simulink model "CH22_3A"  (Simulink 7.5)
settings: Solver=ode45  StartTime=0.0  StopTime=20  RelTol=1e-3
libraries: commrandsrc2 x2, commutil2 x2, commfilt2 x1
settings Model: Creator=my2  LastModifiedBy=xnote
settings OptimizationCC: ExpressionDepthLimit=128
settings DebuggingCC: MultiTaskDSMMsg=warning  MultiTaskCondExecSysMsg=none  StateNameClashWarn=none  StrictBusMsg=None
settings RTWCC: IncludeERTFirstTime=on
settings CodeAppCC: CustomSymbolStrType=$N$R$M_T
settings GRTTargetCC: CombineOutputUpdateFcns=on  CPPClassGenCompliant=on

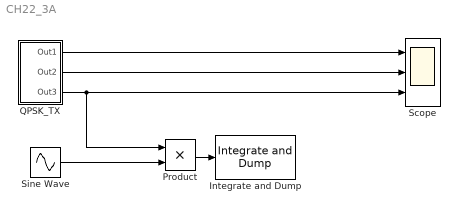
== system CH22_3A ==
  Integrate and Dump : commfilt2/Integrate and Dump  DialogController=commDDGCreate  DialogControllerArgs=DataTag0  obssamples=8  offsetsamples=0  nodump=off  roundingMode=Floor  overflowMode=off
  Product : Product
  QPSK_TX : Subsystem
  Scope : Scope  NumInputPorts=3
      settings: YMin=-5~-5~-5  YMax=5~5~5
  Sine Wave : Sin  Amplitude=1  Bias=0  Frequency=1  Phase=0  Samples=10  SampleTime=1/256  Offset=0
  wires:
  QPSK_TX/1(Out1) -> Scope/1
  QPSK_TX/2(Out2) -> Scope/2
  QPSK_TX/3(Out3) -> Product/1, Scope/3
  Sine Wave/1 -> Product/2
  Product/1 -> Integrate and Dump/1

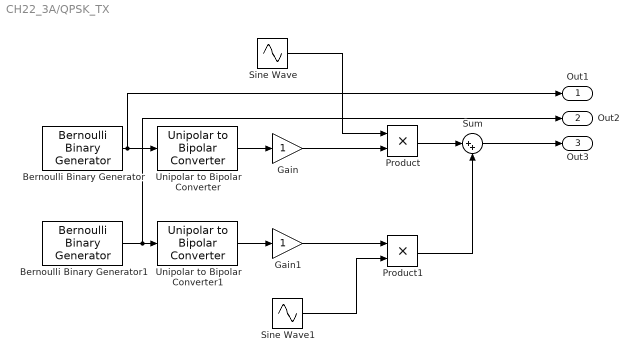
== system CH22_3A/QPSK_TX ==
  Bernoulli Binary Generator : commrandsrc2/Bernoulli Binary Generator  DialogController=commDDGCreate  DialogControllerArgs=DataTag1  SystemSampleTime=-1  P=0.5  seed=71  Ts=1  frameBased=off  sampPerFrame=1  orient=off  outDataType=boolean
  Bernoulli Binary Generator1 : commrandsrc2/Bernoulli Binary Generator  DialogController=commDDGCreate  DialogControllerArgs=DataTag2  SystemSampleTime=-1  P=0.5  seed=61  Ts=1  frameBased=off  sampPerFrame=1  orient=off  outDataType=boolean
  Gain : Gain
  Gain1 : Gain
  Product : Product
  Product1 : Product
  Sine Wave : Sin  Amplitude=1  Bias=0  Frequency=1  Phase=0  Samples=10  SampleTime=1/256  Offset=0
  Sine Wave1 : Sin  Amplitude=1  Bias=0  Frequency=1  Phase=0  Samples=10  SampleTime=1/256  Offset=0
  Sum : Sum  Inputs=|++
  Unipolar to Bipolar Converter : commutil2/Unipolar to Bipolar Converter  SystemSampleTime=-1  M=2  polarity=Positive  dataType=Inherit via internal rule
  Unipolar to Bipolar Converter1 : commutil2/Unipolar to Bipolar Converter  SystemSampleTime=-1  M=2  polarity=Positive  dataType=Inherit via internal rule
  Out1 : Outport
  Out2 : Outport  Port=2
  Out3 : Outport  Port=3
  wires:
  Sum/1 -> Out3/1
  Unipolar to Bipolar Converter/1 -> Gain/1
  Sine Wave1/1 -> Product1/2
  Gain1/1 -> Product1/1
  Sine Wave/1 -> Product/1
  Bernoulli Binary Generator/1 -> Out1/1, Unipolar to Bipolar Converter/1
  Product/1 -> Sum/1
  Product1/1 -> Sum/2
  Unipolar to Bipolar Converter1/1 -> Gain1/1
  Bernoulli Binary Generator1/1 -> Out2/1, Unipolar to Bipolar Converter1/1
  Gain/1 -> Product/2
